simulink library "Wheel_System_Const_R"  (R2018b)
settings: Solver=VariableStepAuto  StartTime=0.0  StopTime=10.0  RelTol=1e-3
settings Model: Creator=Tony  LastModifiedBy=ga69qig

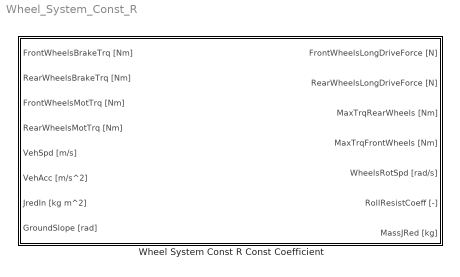
== system Wheel_System_Const_R ==
  Wheel System Const R Const Coefficient : Subsystem  mask(SB){Wheel_Radius=0.3, Wheel_Roll_Resistance=0.009, Wheel_Roll_Resistance_Dyn=0, mu_Tyre=0.7, J_FourWheels=4.96, Gravity=9.81, Wheelbase=1.867, COG_Height=0.5, COG_Front=0.9335, COG_Rear=0.9335, Veh_Mass=1000, LocalSampleTime=-1}
      mask prompts: Wheel_Radius "Wheel Radius [m]"; Wheel_Roll_Resistance "Roll Resistance Coefficient [-]"; Wheel_Roll_Resistance_Dyn "Dynamic Roll Resistance Coefficient [s/m]"; mu_Tyre "Friction Coefficient between Wheel/Road [-]"; J_FourWheels "Inertia Moment of four Wheels [kg m^2]"; Gravity "Gravity [m/s^2]"; Wheelbase "Wheelbase [m]"; COG_Height "Height Center of Gravity over Ground [m]"; COG_Front "Distance from Center of Gravity to Front Axle [m]"; COG_Rear "Distance from Center of Gravity to Rear Axle [m]"; Veh_Mass "Vehicle Mass [kg]"; LocalSampleTime "Local System Sample-Time [s]"
      mask help:
      | <Author> Alexander Koch, Benedikt Danquah based on Stefan Müller [1], Stephan Rohr [2]  </Author>
      | <Date> 15/01/2018 </Date>
      | <Sources>
      | [1] S. Mueller, S. Rohr, und et al, Hrsg, Analysing the Influence of Driver Behaviour and Tuning Measures on Battery Aging and Residual Value of Electric Vehicles, 2017
      | </Sources>
      |
      | <Description>
      | Calculates the longitudinal forces of the front and rear wheels, the rotational speed of the wheels and gives the roll resistant coefficient as an output. There are two roll resistant coefficients. A static parameter and a dynamic one. The dynamic roll resistant coefficient is mutliplied with the velocity and added to the static coefficient. Slip can not be represented. The moment of inertia is transfered to a mass.
      | </Description>
      mask init:
      | GlobalSampleTime = CalcGlobalSampleTime(LocalSampleTime);
      mask Help:
      | <Parameters>
      | Wheel Radius [m]
      | 	<Min> >0 </Min>
      | Roll Resistance Coefficient [-]
      | 	<Min> 0 </Min>
      | Dynamic Roll Resistance Coefficient [s/m]
      | Friction Coefficient between Wheel/Road [-]
      | Inertia Moment of four Wheels [kg m^2]
      | Gravity [m/s^2]
      | Wheelbase [m]
      | Height Center of Gravity over Ground [m]
      | Distance from Center of Gravity to Front Axle [m]
      | Distance from Center of Gravity to Rear Axle [m]
      | Local System Sample-Time [s]
      | 	<Min> GlobalSampleTime </Min>
      | Global Sample-Time [s]
      | </Parameters>
      | 
      | <Inputs>
      | FrontWheelsBrakeTrq [Nm]
      | 	 <sign orientation> [-] results in negative longitudinal driving Force </sign orientation>
      | RearWheelsBrakeTrq [Nm]
      | 	<sign orientation> [-] results in negative longitudinal driving Force </sign orientation>
      | FrontWheelsMotTrq [Nm]
      | 	<sign orientation> [+] results in positive longitudinal driving force </sign orientation>
      | RearWheelsMotTrq [Nm]
      | 	<sign orientation> [+] results in positive longitudinal driving force </sign orientation>
      | VehSpd [m/s]
      | VehAcc [m/s^2]
      | JRedIn [kg m^2]
      | GroundSlope [rad]
      | MassVehicle [kg]
      | </Inputs>
      | 
      | <Outputs>
      | FrontWheelsLongDriveForce [N]
      | RearWheelsLonDriveForce [N]
      | MaxTrqFrontWheels [Nm]
      | MaxTrqRearWheels [Nm]
      | WheelsRotSpd [rad/s]
      | RollResistCoeff [-]
      | MassJRed [kg]
      | </Outputs>
      | <Sources>
      | [1] S. Mueller, S. Rohr, W. Schmid, and M. Lienkamp, “Analysing the Influence of Driver Behaviour and Tuning Measures on Battery Aging and Residual Value of Electric Vehicles,” in Proc. EVS30 Symposium, Stuttgart, 2017, pp. 1–12.
      | [2] S. Rohr, “Technisch-wirtschaftliche Analyse des Zweitnutzungs- potentials von Lithium-Ionen-Traktionsbatterien,” Dissertation, Institute of Automotive Technology, Technical University Munich, Munich, 2018.
      | </Sources>
      mask TypeOptions Wheel_Radius: Wheel_Radius/Value
      mask TypeOptions Wheel_Roll_Resistance: Wheel_Roll_Resistance_Coeff/Value
      mask TypeOptions Wheel_Roll_Resistance_Dyn: Wheel_Roll_Resistance_Coeff_Dyn/Value
      mask TypeOptions mu_Tyre: mu_tyre/Value
      mask TypeOptions J_FourWheels: J_FourWheels/Value
      mask TypeOptions Gravity: Gravity/Value
      mask TypeOptions Wheelbase: Wheelbase/Value
      mask TypeOptions COG_Height: COG_Height/Value
      mask TypeOptions COG_Front: COG_Front/Value
      mask TypeOptions COG_Rear: COG_Rear/Value
      mask TypeOptions Veh_Mass: Vehicle_Mass/Value
      mask TypeOptions LocalSampleTime: FrontWheelsBrakeTrq [Nm]/SampleTime | RearWheelsBrakeTrq [Nm]/SampleTime | FrontWheelsMotTrq [Nm]/SampleTime | RearWheelsMotTrq [Nm]/SampleTime | VehSpd [m//s]/SampleTime | VehAcc [m//s^2]/SampleTime | JredIn [kg m^2]/SampleTime | GroundSlope [rad]/SampleTime
      mask DialogControl Container3 Prompt: Documentation
      mask DialogControl Control2 Prompt: %<MaskHelp>
      mask DialogControl Container5 Prompt: Sample Time
      mask Display:
      | [picturexpos,pictureypos,picturewidth,pictureheight] = ...
      |     CalcBlockPicturePosition(gcb,1,0.01,0.1,120,120); % calculating picture position depending on Block size and minimum margin size
      | image('Wheel_System_Const_R.svg',[picturexpos pictureypos picturewidth pictureheight]); % plot picture to block

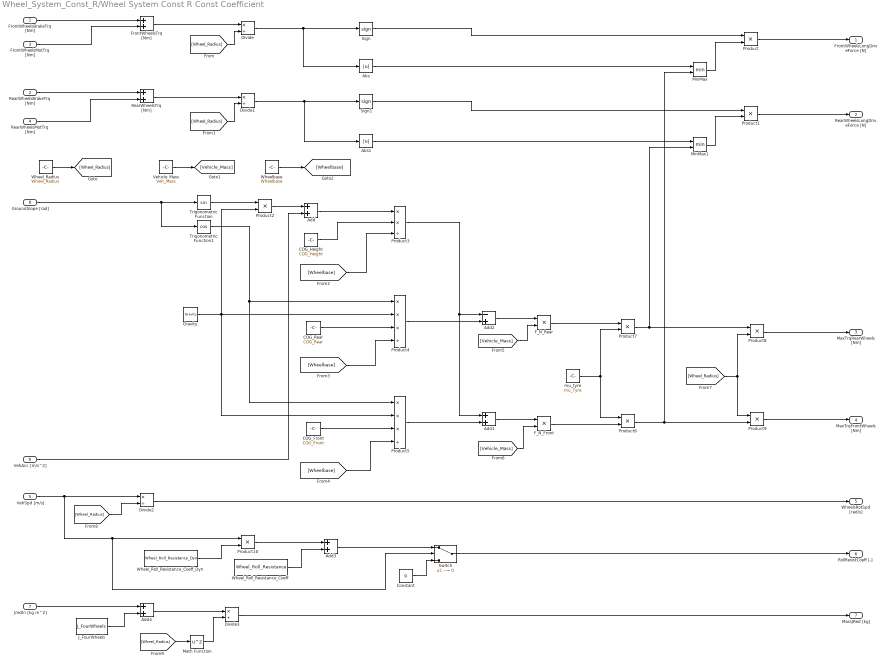
== system Wheel_System_Const_R/Wheel System Const R Const Coefficient ==
  FrontWheelsBrakeTrq [Nm] : Inport  SampleTime=LocalSampleTime
  RearWheelsBrakeTrq [Nm] : Inport  Port=2  SampleTime=LocalSampleTime
  FrontWheelsMotTrq [Nm] : Inport  Port=3  SampleTime=LocalSampleTime
  RearWheelsMotTrq [Nm] : Inport  Port=4  SampleTime=LocalSampleTime
  VehSpd [m/s] : Inport  Port=5  SampleTime=LocalSampleTime
  VehAcc [m/s^2] : Inport  Port=6  SampleTime=LocalSampleTime
  JredIn [kg m^2] : Inport  Port=7  SampleTime=LocalSampleTime
  GroundSlope [rad] : Inport  Port=8  SampleTime=LocalSampleTime
  Abs : Abs
  Abs1 : Abs
  Add{,1,3..4} (4 alike) : Sum
  Add2 : Sum  Inputs=-+
  COG_Front : Constant  Value=COG_Front
  COG_Height : Constant  Value=COG_Height
  COG_Rear : Constant  Value=COG_Rear
  Constant : Constant  Value=0
  Divide{,1..3} (4 alike) : Product  Inputs=*/
  F_N_Front : Product
  F_N_Rear : Product
  FrontWheelsTrq [Nm] : Sum
  Gravity : Constant  Value=Gravity
  J_FourWheels : Constant  Value=J_FourWheels
  Math Function : Math  Operator=square  SaturateOnIntegerOverflow=on
  MinMax : MinMax  Inputs=2
  MinMax1 : MinMax  Inputs=2
  Product{,1..2,6..10} (8 alike) : Product
  Product3 : Product  Inputs=**/
  Product4 : Product  Inputs=***/
  Product5 : Product  Inputs=***/
  RearWheelsTrq [Nm] : Sum
  Sign : Signum
  Sign1 : Signum
  Switch : Switch  Criteria=u2 ~= 0
  Trigonometric Function : Trigonometry
  Trigonometric Function1 : Trigonometry  Operator=cos
  Vehicle_Mass : Constant  Value=Veh_Mass
  Wheel_Radius : Constant  Value=Wheel_Radius
  Wheel_Roll_Resistance_Coeff : Constant  Value=Wheel_Roll_Resistance
  Wheel_Roll_Resistance_Coeff_Dyn : Constant  Value=Wheel_Roll_Resistance_Dyn
  Wheelbase : Constant  Value=Wheelbase
  mu_tyre : Constant  Value=mu_Tyre
  FrontWheelsLongDriveForce [N] : Outport  SampleTime=GlobalSampleTime
  RearWheelsLongDriveForce [N] : Outport  Port=2  SampleTime=GlobalSampleTime
  MaxTrqRearWheels [Nm] : Outport  Port=3  SampleTime=GlobalSampleTime
  MaxTrqFrontWheels [Nm] : Outport  Port=4  SampleTime=GlobalSampleTime
  WheelsRotSpd [rad/s] : Outport  Port=5  SampleTime=GlobalSampleTime
  RollResistCoeff [-] : Outport  Port=6  SampleTime=GlobalSampleTime
  MassJRed [kg] : Outport  Port=7  SampleTime=GlobalSampleTime
  wires:
  FrontWheelsBrakeTrq [Nm]/1 -> FrontWheelsTrq [Nm]/1
  FrontWheelsMotTrq [Nm]/1 -> FrontWheelsTrq [Nm]/2
  RearWheelsBrakeTrq [Nm]/1 -> RearWheelsTrq [Nm]/1
  RearWheelsMotTrq [Nm]/1 -> RearWheelsTrq [Nm]/2
  FrontWheelsTrq [Nm]/1 -> Divide/1
  RearWheelsTrq [Nm]/1 -> Divide1/1
  Product/1 -> FrontWheelsLongDriveForce [N]/1
  Sign/1 -> Product/1
  Divide/1 -> Abs/1, Sign/1
  Abs/1 -> MinMax/1
  MinMax/1 -> Product/2
  Wheel_Radius/1 -> [Wheel_Radius]
  [Wheel_Radius] -> Divide/2
  [Wheel_Radius] -> Divide1/2
  Divide1/1 -> Abs1/1, Sign1/1
  Abs1/1 -> MinMax1/1
  Sign1/1 -> Product1/1
  MinMax1/1 -> Product1/2
  Product1/1 -> RearWheelsLongDriveForce [N]/1
  Vehicle_Mass/1 -> [Vehicle_Mass]
  GroundSlope [rad]/1 -> Trigonometric Function1/1, Trigonometric Function/1
  Trigonometric Function/1 -> Product2/1
  Product2/1 -> Add/1
  VehAcc [m/s^2]/1 -> Add/2
  Add/1 -> Product3/1
  COG_Height/1 -> Product3/2
  Trigonometric Function1/1 -> Product4/1, Product5/1
  Gravity/1 -> Product2/2, Product5/2, Product4/2
  COG_Rear/1 -> Product4/3
  Wheelbase/1 -> [Wheelbase]
  [Wheelbase] -> Product3/3
  [Wheelbase] -> Product4/4
  COG_Front/1 -> Product5/3
  [Wheelbase] -> Product5/4
  Product5/1 -> Add1/2
  Product3/1 -> Add2/1, Add1/1
  Product4/1 -> Add2/2
  Add2/1 -> F_N_Rear/1
  Add1/1 -> F_N_Front/1
  [Vehicle_Mass] -> F_N_Rear/2
  [Vehicle_Mass] -> F_N_Front/2
  F_N_Rear/1 -> Product7/1
  F_N_Front/1 -> Product6/2
  mu_tyre/1 -> Product6/1, Product7/2
  Product6/1 -> Product9/2, MinMax/2
  Product7/1 -> Product8/1, MinMax1/2
  [Wheel_Radius] -> Product8/2, Product9/1
  Product8/1 -> MaxTrqRearWheels [Nm]/1
  Product9/1 -> MaxTrqFrontWheels [Nm]/1
  VehSpd [m/s]/1 -> Switch/2, Product10/1, Divide2/1
  [Wheel_Radius] -> Divide2/2
  Divide2/1 -> WheelsRotSpd [rad/s]/1
  Wheel_Roll_Resistance_Coeff_Dyn/1 -> Product10/2
  Product10/1 -> Add3/1
  Wheel_Roll_Resistance_Coeff/1 -> Add3/2
  Add3/1 -> Switch/1
  Constant/1 -> Switch/3
  Switch/1 -> RollResistCoeff [-]/1
  JredIn [kg m^2]/1 -> Add4/1
  J_FourWheels/1 -> Add4/2
  Add4/1 -> Divide3/1
  Math Function/1 -> Divide3/2
  [Wheel_Radius] -> Math Function/1
  Divide3/1 -> MassJRed [kg]/1
